simulink model "MultirotorModel_Debugging"  (R2025b)
settings: Solver=ode4  StartTime=0.0  StopTime=350  FixedStep=0.005  RelTol=1e-3  EnableMultiTasking=on
undefined symbols (not defined in the file): angControlTuning, angRateControlTuning, bounds, Controller, decyear, DiscIntNeverNeededParam, DroneMass, dyn_obs, Dz, Gravity, initialConditions, initialGainsMultiplier, Iz, leapyear, max_deviazione_pos, num_rays, Nz, pos_goal, posControlTuning, Pz, startFlightTime, tolleranza_goal, tunePositionController, UAVSampleTime, Vehicle, velControlTuning
libraries: slpidlib x37, slctrl_autotuning x25, sharedutil x4, aerolibconvert2 x3, aerolibatmos2 x2, aerolibgravity2 x2, shared6dof x2, aerolibasang x2, sensorinslib x2, matrix_library x1, uavutilslib x1, uavalgslib x1
(part 6 of 8)

== system MultirotorModel_Debugging/Inner Loop and Plant Model/High-FidelityModel/Control System/Controller/Attitude Controller (autotuning)/Angular Velocity Loop Autotuning ==
  AngVelCtrl_out : Inport
  pitchrollrate_fdbk : Inport  Port=2
  Closed-Loop PID Autotuner : slctrl_autotuning/Closed-Loop PID Autotuner  PIDType=PIDF  PIDForm=Parallel  TimeDomain=discrete-time  DiscreteTs=UAVSampleTime  TuningTs=0.2  UseTuningTs=off  IntegratorFormula=Forward Euler  FilterFormula=Forward Euler  ContinuousTs=0.02  Bandwidth=angRateControlTuning.wc  UseExternalWC=off  TargetPM=angRateControlTuning.pm  UseExternalPM=off  UseExternalAchievedPM=off  ExperimentMode=Superposition  PlantType=Stable  PlantSign=Positive  AmpSine=angRateControlTuning.sineAmp  UseExternalAmpSine=off  UseExternalFRD=off  UseExternalU0=off  UseCompanion=off  NotDeployTuningModule=off  UsePLCCoder=off  OutputMode=perturbation only  BlockDataType=single  UseExperimentGoodPort=off  UseConnectedPID=on  blockpath=[]  tunedP=0  tunedI=0  tunedD=0  tunedN=100  tunedPM=0  EstimationWindowSize=3  UseExternalTuningParams=off  SingleMultiRateVariant=SingleSamplingRate  NumEstimationPeriods=4  NumSettlingPeriods=2  NumOfPRBSPeriod=1  PRBSSignalOrder=12  ExperimentModeVariant=VariantSuperimposed  OutputChoice=VariantDonly  ConvergenceCalcVariant=ConvSuperpositionPRBSVariant
  Closed-Loop PID Autotuner1 : slctrl_autotuning/Closed-Loop PID Autotuner  PIDType=PIDF  PIDForm=Parallel  TimeDomain=discrete-time  DiscreteTs=UAVSampleTime  TuningTs=0.2  UseTuningTs=off  IntegratorFormula=Forward Euler  FilterFormula=Forward Euler  ContinuousTs=0.02  Bandwidth=angRateControlTuning.wc  UseExternalWC=off  TargetPM=angRateControlTuning.pm  UseExternalPM=off  UseExternalAchievedPM=off  ExperimentMode=Superposition  PlantType=Stable  PlantSign=Positive  AmpSine=angRateControlTuning.sineAmp  UseExternalAmpSine=off  UseExternalFRD=off  UseExternalU0=off  UseCompanion=off  NotDeployTuningModule=off  UsePLCCoder=off  OutputMode=perturbation only  BlockDataType=single  UseExperimentGoodPort=off  UseConnectedPID=on  blockpath=[]  tunedP=0  tunedI=0  tunedD=0  tunedN=100  tunedPM=0  EstimationWindowSize=3  UseExternalTuningParams=off  SingleMultiRateVariant=SingleSamplingRate  NumEstimationPeriods=4  NumSettlingPeriods=2  NumOfPRBSPeriod=1  PRBSSignalOrder=12  ExperimentModeVariant=VariantSuperimposed  OutputChoice=VariantDonly  ConvergenceCalcVariant=ConvSuperpositionPRBSVariant
  Display : Display
  Display1 : Display
  Mux : Mux  Inputs=2
  Scope : Scope
      settings: ActiveDisplayYMinimum=99.18257  ActiveDisplayYMaximum=100.62707  DataLoggingVariableName=ScopeData9
  Scope1 : Scope
      settings: DataLoggingVariableName=ScopeData10
  Selector : Selector  InputPortWidth=2  IndexOptions=Index vector (dialog)  Indices=1  OutputSizes=1
  Selector1 : Selector  InputPortWidth=2  IndexOptions=Index vector (dialog)  Indices=1  OutputSizes=1
  Selector2 : Selector  InputPortWidth=2  IndexOptions=Index vector (dialog)  Indices=2  OutputSizes=1
  Selector3 : Selector  InputPortWidth=2  IndexOptions=Index vector (dialog)  Indices=2  OutputSizes=1
  Step : Step  Time=angRateControlTuning.startExpRoll  SampleTime=UAVSampleTime
  Step1 : Step  Time=angRateControlTuning.stopExpRoll  After=-1  SampleTime=UAVSampleTime
  Step2 : Step  Time=angRateControlTuning.startExpPitch  SampleTime=UAVSampleTime
  Step3 : Step  Time=angRateControlTuning.stopExpPitch  After=-1  SampleTime=UAVSampleTime
  Sum : Sum  Inputs=|++
  Sum1 : Sum  Inputs=|++
  Update PID Gains : Subsystem
  pitchrollrate_perturb : Outport
  wires:
  Closed-Loop PID Autotuner1/1 -> Mux/2
  Closed-Loop PID Autotuner1/2 -> Scope1/1
  Sum1/1 -> Update PID Gains/3(start/stop rollrate), Closed-Loop PID Autotuner1/3
  Step/1 -> Sum1/1
  Step1/1 -> Sum1/2
  Selector3/1 -> Closed-Loop PID Autotuner1/2
  Selector2/1 -> Closed-Loop PID Autotuner1/1
  Closed-Loop PID Autotuner/1 -> Mux/1
  Mux/1 -> pitchrollrate_perturb/1
  Closed-Loop PID Autotuner/2 -> Scope/1
  Step3/1 -> Sum/2
  Step2/1 -> Sum/1
  Sum/1 -> Update PID Gains/2(start/stop pitchrate), Closed-Loop PID Autotuner/3
  Selector1/1 -> Closed-Loop PID Autotuner/2
  Selector/1 -> Closed-Loop PID Autotuner/1
  pitchrollrate_fdbk/1 -> Selector1/1, Selector3/1
  AngVelCtrl_out/1 -> Selector/1, Selector2/1
  Closed-Loop PID Autotuner/3 -> Update PID Gains/1(PID Gains pitchrate), Display/1
  Closed-Loop PID Autotuner1/3 -> Update PID Gains/4(PID Gains rollrate), Display1/1

== system MultirotorModel_Debugging/Inner Loop and Plant Model/High-FidelityModel/Control System/Controller/Position Controller (autotuning)/Position Loop Autotuning ==
  PosCtrl_out : Inport
  xy_fdbk : Inport  Port=2
  Closed-Loop PID Autotuner : slctrl_autotuning/Closed-Loop PID Autotuner  PIDType=P  PIDForm=Parallel  TimeDomain=discrete-time  DiscreteTs=UAVSampleTime  TuningTs=0.2  UseTuningTs=off  IntegratorFormula=Forward Euler  FilterFormula=Forward Euler  ContinuousTs=0.02  Bandwidth=posControlTuning.wc  UseExternalWC=off  TargetPM=posControlTuning.pm  UseExternalPM=off  UseExternalAchievedPM=off  ExperimentMode=Superposition  PlantType=Stable  PlantSign=Positive  AmpSine=posControlTuning.sineAmp  UseExternalAmpSine=off  UseExternalFRD=off  UseExternalU0=off  UseCompanion=off  NotDeployTuningModule=off  UsePLCCoder=off  OutputMode=perturbation only  BlockDataType=single  UseExperimentGoodPort=off  UseConnectedPID=on  blockpath=[]  tunedP=0  tunedI=0  tunedD=0  tunedN=100  tunedPM=0  EstimationWindowSize=3  UseExternalTuningParams=off  SingleMultiRateVariant=SingleSamplingRate  NumEstimationPeriods=4  NumSettlingPeriods=2  NumOfPRBSPeriod=1  PRBSSignalOrder=12  ExperimentModeVariant=VariantSuperimposed  OutputChoice=VariantDonly  ConvergenceCalcVariant=ConvSuperpositionPRBSVariant
  Closed-Loop PID Autotuner1 : slctrl_autotuning/Closed-Loop PID Autotuner  PIDType=P  PIDForm=Parallel  TimeDomain=discrete-time  DiscreteTs=UAVSampleTime  TuningTs=0.2  UseTuningTs=off  IntegratorFormula=Forward Euler  FilterFormula=Forward Euler  ContinuousTs=0.02  Bandwidth=posControlTuning.wc  UseExternalWC=off  TargetPM=posControlTuning.pm  UseExternalPM=off  UseExternalAchievedPM=off  ExperimentMode=Superposition  PlantType=Stable  PlantSign=Positive  AmpSine=posControlTuning.sineAmp  UseExternalAmpSine=off  UseExternalFRD=off  UseExternalU0=off  UseCompanion=off  NotDeployTuningModule=off  UsePLCCoder=off  OutputMode=perturbation only  BlockDataType=single  UseExperimentGoodPort=off  UseConnectedPID=on  blockpath=[]  tunedP=0  tunedI=0  tunedD=0  tunedN=100  tunedPM=0  EstimationWindowSize=3  UseExternalTuningParams=off  SingleMultiRateVariant=SingleSamplingRate  NumEstimationPeriods=4  NumSettlingPeriods=2  NumOfPRBSPeriod=1  PRBSSignalOrder=12  ExperimentModeVariant=VariantSuperimposed  OutputChoice=VariantDonly  ConvergenceCalcVariant=ConvSuperpositionPRBSVariant
  Display : Display
  Display1 : Display
  Gain1 : Gain  Gain=tunePositionController
  Gain2 : Gain  Gain=tunePositionController
  Mux : Mux  Inputs=2
  Selector : Selector  InputPortWidth=2  IndexOptions=Index vector (dialog)  Indices=1  OutputSizes=1
  Selector1 : Selector  InputPortWidth=2  IndexOptions=Index vector (dialog)  Indices=1  OutputSizes=1
  Selector2 : Selector  InputPortWidth=2  IndexOptions=Index vector (dialog)  Indices=2  OutputSizes=1
  Selector3 : Selector  InputPortWidth=2  IndexOptions=Index vector (dialog)  Indices=2  OutputSizes=1
  Step : Step  Time=posControlTuning.startExpX  SampleTime=UAVSampleTime
  Step1 : Step  Time=posControlTuning.stopExpX  After=-1  SampleTime=UAVSampleTime
  Step2 : Step  Time=posControlTuning.startExpY  SampleTime=UAVSampleTime
  Step3 : Step  Time=posControlTuning.stopExpY  After=-1  SampleTime=UAVSampleTime
  Sum : Sum  Inputs=|++
  Sum1 : Sum  Inputs=|++
  Terminator : Terminator
  Terminator1 : Terminator
  Update PID Gains : Subsystem
  xy_perturb : Outport
  wires:
  PosCtrl_out/1 -> Selector2/1, Selector/1
  xy_fdbk/1 -> Selector3/1, Selector1/1
  Selector/1 -> Closed-Loop PID Autotuner/1
  Selector1/1 -> Closed-Loop PID Autotuner/2
  Sum/1 -> Gain1/1
  Step/1 -> Sum/1
  Step1/1 -> Sum/2
  Closed-Loop PID Autotuner/2 -> Terminator/1
  Mux/1 -> xy_perturb/1
  Closed-Loop PID Autotuner/1 -> Mux/1
  Selector2/1 -> Closed-Loop PID Autotuner1/1
  Selector3/1 -> Closed-Loop PID Autotuner1/2
  Step3/1 -> Sum1/2
  Step2/1 -> Sum1/1
  Sum1/1 -> Gain2/1
  Closed-Loop PID Autotuner1/2 -> Terminator1/1
  Closed-Loop PID Autotuner1/1 -> Mux/2
  Closed-Loop PID Autotuner/3 -> Update PID Gains/1(PID Gains X), Display/1
  Closed-Loop PID Autotuner1/3 -> Update PID Gains/4(PID Gains Y), Display1/1
  Gain1/1 -> Update PID Gains/2(start/stop X), Closed-Loop PID Autotuner/3
  Gain2/1 -> Update PID Gains/3(start/stop Y), Closed-Loop PID Autotuner1/3

== system MultirotorModel_Debugging/Inner Loop and Plant Model/High-FidelityModel/Control System/Controller/Position Controller (autotuning)/Velocity Loop Autotuning ==
  VelCtrl_out : Inport
  xxyy_fdbk : Inport  Port=2
  Closed-Loop PID Autotuner : slctrl_autotuning/Closed-Loop PID Autotuner  PIDType=PI  PIDForm=Parallel  TimeDomain=discrete-time  DiscreteTs=UAVSampleTime  TuningTs=0.2  UseTuningTs=off  IntegratorFormula=Forward Euler  FilterFormula=Forward Euler  ContinuousTs=0.02  Bandwidth=velControlTuning.wc  UseExternalWC=off  TargetPM=velControlTuning.pm  UseExternalPM=off  UseExternalAchievedPM=off  ExperimentMode=Superposition  PlantType=Stable  PlantSign=Positive  AmpSine=velControlTuning.sineAmp  UseExternalAmpSine=off  UseExternalFRD=off  UseExternalU0=off  UseCompanion=off  NotDeployTuningModule=off  UsePLCCoder=off  OutputMode=perturbation only  BlockDataType=single  UseExperimentGoodPort=off  UseConnectedPID=on  blockpath=[]  tunedP=0  tunedI=0  tunedD=0  tunedN=100  tunedPM=0  EstimationWindowSize=3  UseExternalTuningParams=off  SingleMultiRateVariant=SingleSamplingRate  NumEstimationPeriods=4  NumSettlingPeriods=2  NumOfPRBSPeriod=1  PRBSSignalOrder=12  ExperimentModeVariant=VariantSuperimposed  OutputChoice=VariantDonly  ConvergenceCalcVariant=ConvSuperpositionPRBSVariant
  Closed-Loop PID Autotuner1 : slctrl_autotuning/Closed-Loop PID Autotuner  PIDType=PI  PIDForm=Parallel  TimeDomain=discrete-time  DiscreteTs=UAVSampleTime  TuningTs=0.2  UseTuningTs=off  IntegratorFormula=Forward Euler  FilterFormula=Forward Euler  ContinuousTs=0.02  Bandwidth=velControlTuning.wc  UseExternalWC=off  TargetPM=velControlTuning.pm  UseExternalPM=off  UseExternalAchievedPM=off  ExperimentMode=Superposition  PlantType=Stable  PlantSign=Positive  AmpSine=velControlTuning.sineAmp  UseExternalAmpSine=off  UseExternalFRD=off  UseExternalU0=off  UseCompanion=off  NotDeployTuningModule=off  UsePLCCoder=off  OutputMode=perturbation only  BlockDataType=single  UseExperimentGoodPort=off  UseConnectedPID=on  blockpath=[]  tunedP=0  tunedI=0  tunedD=0  tunedN=100  tunedPM=0  EstimationWindowSize=3  UseExternalTuningParams=off  SingleMultiRateVariant=SingleSamplingRate  NumEstimationPeriods=4  NumSettlingPeriods=2  NumOfPRBSPeriod=1  PRBSSignalOrder=12  ExperimentModeVariant=VariantSuperimposed  OutputChoice=VariantDonly  ConvergenceCalcVariant=ConvSuperpositionPRBSVariant
  Display : Display
  Display1 : Display
  Gain : Gain  Gain=tunePositionController
  Gain1 : Gain  Gain=tunePositionController
  Mux : Mux  Inputs=2
  Scope : Scope
      settings: ActiveDisplayYMinimum=99.18257  ActiveDisplayYMaximum=100.62707  DataLoggingVariableName=ScopeData9
  Scope1 : Scope
      settings: DataLoggingVariableName=ScopeData10
  Selector : Selector  InputPortWidth=2  IndexOptions=Index vector (dialog)  Indices=1  OutputSizes=1
  Selector1 : Selector  InputPortWidth=2  IndexOptions=Index vector (dialog)  Indices=1  OutputSizes=1
  Selector2 : Selector  InputPortWidth=2  IndexOptions=Index vector (dialog)  Indices=2  OutputSizes=1
  Selector3 : Selector  InputPortWidth=2  IndexOptions=Index vector (dialog)  Indices=2  OutputSizes=1
  Step : Step  Time=velControlTuning.startExpX  SampleTime=UAVSampleTime
  Step1 : Step  Time=velControlTuning.stopExpX  After=-1  SampleTime=UAVSampleTime
  Step2 : Step  Time=velControlTuning.startExpY  SampleTime=UAVSampleTime
  Step3 : Step  Time=velControlTuning.stopExpY  After=-1  SampleTime=UAVSampleTime
  Sum : Sum  Inputs=|++
  Sum1 : Sum  Inputs=|++
  Update PID Gains : Subsystem
  xxyy_perturb : Outport
  wires:
  Closed-Loop PID Autotuner1/1 -> Mux/2
  Closed-Loop PID Autotuner1/2 -> Scope1/1
  Sum1/1 -> Gain1/1
  Step2/1 -> Sum1/1
  Step3/1 -> Sum1/2
  Selector3/1 -> Closed-Loop PID Autotuner1/2
  Selector2/1 -> Closed-Loop PID Autotuner1/1
  Closed-Loop PID Autotuner/1 -> Mux/1
  Mux/1 -> xxyy_perturb/1
  Closed-Loop PID Autotuner/2 -> Scope/1
  Step1/1 -> Sum/2
  Step/1 -> Sum/1
  Sum/1 -> Gain/1
  Selector1/1 -> Closed-Loop PID Autotuner/2
  Selector/1 -> Closed-Loop PID Autotuner/1
  xxyy_fdbk/1 -> Selector1/1, Selector3/1
  VelCtrl_out/1 -> Selector/1, Selector2/1
  Closed-Loop PID Autotuner/3 -> Update PID Gains/1(PID Gains XX), Display/1
  Closed-Loop PID Autotuner1/3 -> Update PID Gains/4(PID Gains YY), Display1/1
  Gain/1 -> Update PID Gains/2(start/stop XX), Closed-Loop PID Autotuner/3
  Gain1/1 -> Update PID Gains/3(start/stop YY), Closed-Loop PID Autotuner1/3

== system MultirotorModel_Debugging/Inner Loop and Plant Model/High-FidelityModel/Control System/Controller/Position Controller (autotuning, solo vel)/Position Loop Autotuning ==
  PosCtrl_out : Inport
  xy_fdbk : Inport  Port=2
  Closed-Loop PID Autotuner : slctrl_autotuning/Closed-Loop PID Autotuner  PIDType=P  PIDForm=Parallel  TimeDomain=discrete-time  DiscreteTs=UAVSampleTime  TuningTs=0.2  UseTuningTs=off  IntegratorFormula=Forward Euler  FilterFormula=Forward Euler  ContinuousTs=0.02  Bandwidth=posControlTuning.wc  UseExternalWC=off  TargetPM=posControlTuning.pm  UseExternalPM=off  UseExternalAchievedPM=off  ExperimentMode=Superposition  PlantType=Stable  PlantSign=Positive  AmpSine=posControlTuning.sineAmp  UseExternalAmpSine=off  UseExternalFRD=off  UseExternalU0=off  UseCompanion=off  NotDeployTuningModule=off  UsePLCCoder=off  OutputMode=perturbation only  BlockDataType=single  UseExperimentGoodPort=off  UseConnectedPID=on  blockpath=[]  tunedP=0  tunedI=0  tunedD=0  tunedN=100  tunedPM=0  EstimationWindowSize=3  UseExternalTuningParams=off  SingleMultiRateVariant=SingleSamplingRate  NumEstimationPeriods=4  NumSettlingPeriods=2  NumOfPRBSPeriod=1  PRBSSignalOrder=12  ExperimentModeVariant=VariantSuperimposed  OutputChoice=VariantDonly  ConvergenceCalcVariant=ConvSuperpositionPRBSVariant
  Closed-Loop PID Autotuner1 : slctrl_autotuning/Closed-Loop PID Autotuner  PIDType=P  PIDForm=Parallel  TimeDomain=discrete-time  DiscreteTs=UAVSampleTime  TuningTs=0.2  UseTuningTs=off  IntegratorFormula=Forward Euler  FilterFormula=Forward Euler  ContinuousTs=0.02  Bandwidth=posControlTuning.wc  UseExternalWC=off  TargetPM=posControlTuning.pm  UseExternalPM=off  UseExternalAchievedPM=off  ExperimentMode=Superposition  PlantType=Stable  PlantSign=Positive  AmpSine=posControlTuning.sineAmp  UseExternalAmpSine=off  UseExternalFRD=off  UseExternalU0=off  UseCompanion=off  NotDeployTuningModule=off  UsePLCCoder=off  OutputMode=perturbation only  BlockDataType=single  UseExperimentGoodPort=off  UseConnectedPID=on  blockpath=[]  tunedP=0  tunedI=0  tunedD=0  tunedN=100  tunedPM=0  EstimationWindowSize=3  UseExternalTuningParams=off  SingleMultiRateVariant=SingleSamplingRate  NumEstimationPeriods=4  NumSettlingPeriods=2  NumOfPRBSPeriod=1  PRBSSignalOrder=12  ExperimentModeVariant=VariantSuperimposed  OutputChoice=VariantDonly  ConvergenceCalcVariant=ConvSuperpositionPRBSVariant
  Display : Display
  Display1 : Display
  Gain1 : Gain  Gain=tunePositionController
  Gain2 : Gain  Gain=tunePositionController
  Mux : Mux  Inputs=2
  Selector : Selector  InputPortWidth=2  IndexOptions=Index vector (dialog)  Indices=1  OutputSizes=1
  Selector1 : Selector  InputPortWidth=2  IndexOptions=Index vector (dialog)  Indices=1  OutputSizes=1
  Selector2 : Selector  InputPortWidth=2  IndexOptions=Index vector (dialog)  Indices=2  OutputSizes=1
  Selector3 : Selector  InputPortWidth=2  IndexOptions=Index vector (dialog)  Indices=2  OutputSizes=1
  Step : Step  Time=posControlTuning.startExpX  SampleTime=UAVSampleTime
  Step1 : Step  Time=posControlTuning.stopExpX  After=-1  SampleTime=UAVSampleTime
  Step2 : Step  Time=posControlTuning.startExpY  SampleTime=UAVSampleTime
  Step3 : Step  Time=posControlTuning.stopExpY  After=-1  SampleTime=UAVSampleTime
  Sum : Sum  Inputs=|++
  Sum1 : Sum  Inputs=|++
  Terminator : Terminator
  Terminator1 : Terminator
  Update PID Gains : Subsystem
  xy_perturb : Outport
  wires:
  PosCtrl_out/1 -> Selector2/1, Selector/1
  xy_fdbk/1 -> Selector3/1, Selector1/1
  Selector/1 -> Closed-Loop PID Autotuner/1
  Selector1/1 -> Closed-Loop PID Autotuner/2
  Sum/1 -> Gain1/1
  Step/1 -> Sum/1
  Step1/1 -> Sum/2
  Closed-Loop PID Autotuner/2 -> Terminator/1
  Mux/1 -> xy_perturb/1
  Closed-Loop PID Autotuner/1 -> Mux/1
  Selector2/1 -> Closed-Loop PID Autotuner1/1
  Selector3/1 -> Closed-Loop PID Autotuner1/2
  Step3/1 -> Sum1/2
  Step2/1 -> Sum1/1
  Sum1/1 -> Gain2/1
  Closed-Loop PID Autotuner1/2 -> Terminator1/1
  Closed-Loop PID Autotuner1/1 -> Mux/2
  Closed-Loop PID Autotuner/3 -> Update PID Gains/1(PID Gains X), Display/1
  Closed-Loop PID Autotuner1/3 -> Update PID Gains/4(PID Gains Y), Display1/1
  Gain1/1 -> Update PID Gains/2(start/stop X), Closed-Loop PID Autotuner/3
  Gain2/1 -> Update PID Gains/3(start/stop Y), Closed-Loop PID Autotuner1/3

== system MultirotorModel_Debugging/Inner Loop and Plant Model/High-FidelityModel/Control System/Controller/Position Controller (autotuning, solo vel)/Velocity Loop Autotuning ==
  VelCtrl_out : Inport
  xxyy_fdbk : Inport  Port=2
  Closed-Loop PID Autotuner : slctrl_autotuning/Closed-Loop PID Autotuner  PIDType=PI  PIDForm=Parallel  TimeDomain=discrete-time  DiscreteTs=UAVSampleTime  TuningTs=0.2  UseTuningTs=off  IntegratorFormula=Forward Euler  FilterFormula=Forward Euler  ContinuousTs=0.02  Bandwidth=velControlTuning.wc  UseExternalWC=off  TargetPM=velControlTuning.pm  UseExternalPM=off  UseExternalAchievedPM=off  ExperimentMode=Superposition  PlantType=Stable  PlantSign=Positive  AmpSine=velControlTuning.sineAmp  UseExternalAmpSine=off  UseExternalFRD=off  UseExternalU0=off  UseCompanion=off  NotDeployTuningModule=off  UsePLCCoder=off  OutputMode=perturbation only  BlockDataType=single  UseExperimentGoodPort=off  UseConnectedPID=on  blockpath=[]  tunedP=0  tunedI=0  tunedD=0  tunedN=100  tunedPM=0  EstimationWindowSize=3  UseExternalTuningParams=off  SingleMultiRateVariant=SingleSamplingRate  NumEstimationPeriods=4  NumSettlingPeriods=2  NumOfPRBSPeriod=1  PRBSSignalOrder=12  ExperimentModeVariant=VariantSuperimposed  OutputChoice=VariantDonly  ConvergenceCalcVariant=ConvSuperpositionPRBSVariant
  Closed-Loop PID Autotuner1 : slctrl_autotuning/Closed-Loop PID Autotuner  PIDType=PI  PIDForm=Parallel  TimeDomain=discrete-time  DiscreteTs=UAVSampleTime  TuningTs=0.2  UseTuningTs=off  IntegratorFormula=Forward Euler  FilterFormula=Forward Euler  ContinuousTs=0.02  Bandwidth=velControlTuning.wc  UseExternalWC=off  TargetPM=velControlTuning.pm  UseExternalPM=off  UseExternalAchievedPM=off  ExperimentMode=Superposition  PlantType=Stable  PlantSign=Positive  AmpSine=velControlTuning.sineAmp  UseExternalAmpSine=off  UseExternalFRD=off  UseExternalU0=off  UseCompanion=off  NotDeployTuningModule=off  UsePLCCoder=off  OutputMode=perturbation only  BlockDataType=single  UseExperimentGoodPort=off  UseConnectedPID=on  blockpath=[]  tunedP=0  tunedI=0  tunedD=0  tunedN=100  tunedPM=0  EstimationWindowSize=3  UseExternalTuningParams=off  SingleMultiRateVariant=SingleSamplingRate  NumEstimationPeriods=4  NumSettlingPeriods=2  NumOfPRBSPeriod=1  PRBSSignalOrder=12  ExperimentModeVariant=VariantSuperimposed  OutputChoice=VariantDonly  ConvergenceCalcVariant=ConvSuperpositionPRBSVariant
  Display : Display
  Display1 : Display
  Gain : Gain  Gain=tunePositionController
  Gain1 : Gain  Gain=tunePositionController
  Mux : Mux  Inputs=2
  Scope : Scope
      settings: ActiveDisplayYMinimum=99.18257  ActiveDisplayYMaximum=100.62707  DataLoggingVariableName=ScopeData9
  Scope1 : Scope
      settings: DataLoggingVariableName=ScopeData10
  Selector : Selector  InputPortWidth=2  IndexOptions=Index vector (dialog)  Indices=1  OutputSizes=1
  Selector1 : Selector  InputPortWidth=2  IndexOptions=Index vector (dialog)  Indices=1  OutputSizes=1
  Selector2 : Selector  InputPortWidth=2  IndexOptions=Index vector (dialog)  Indices=2  OutputSizes=1
  Selector3 : Selector  InputPortWidth=2  IndexOptions=Index vector (dialog)  Indices=2  OutputSizes=1
  Step : Step  Time=velControlTuning.startExpX  SampleTime=UAVSampleTime
  Step1 : Step  Time=velControlTuning.stopExpX  After=-1  SampleTime=UAVSampleTime
  Step2 : Step  Time=velControlTuning.startExpY  SampleTime=UAVSampleTime
  Step3 : Step  Time=velControlTuning.stopExpY  After=-1  SampleTime=UAVSampleTime
  Sum : Sum  Inputs=|++
  Sum1 : Sum  Inputs=|++
  Update PID Gains : Subsystem
  xxyy_perturb : Outport
  wires:
  Closed-Loop PID Autotuner1/1 -> Mux/2
  Closed-Loop PID Autotuner1/2 -> Scope1/1
  Sum1/1 -> Gain1/1
  Step2/1 -> Sum1/1
  Step3/1 -> Sum1/2
  Selector3/1 -> Closed-Loop PID Autotuner1/2
  Selector2/1 -> Closed-Loop PID Autotuner1/1
  Closed-Loop PID Autotuner/1 -> Mux/1
  Mux/1 -> xxyy_perturb/1
  Closed-Loop PID Autotuner/2 -> Scope/1
  Step1/1 -> Sum/2
  Step/1 -> Sum/1
  Sum/1 -> Gain/1
  Selector1/1 -> Closed-Loop PID Autotuner/2
  Selector/1 -> Closed-Loop PID Autotuner/1
  xxyy_fdbk/1 -> Selector1/1, Selector3/1
  VelCtrl_out/1 -> Selector/1, Selector2/1
  Closed-Loop PID Autotuner/3 -> Update PID Gains/1(PID Gains XX), Display/1
  Closed-Loop PID Autotuner1/3 -> Update PID Gains/4(PID Gains YY), Display1/1
  Gain/1 -> Update PID Gains/2(start/stop XX), Closed-Loop PID Autotuner/3
  Gain1/1 -> Update PID Gains/3(start/stop YY), Closed-Loop PID Autotuner1/3

== system MultirotorModel_Debugging/Inner Loop and Plant Model/High-FidelityModel/Control System/Controller/Position Controller 3 (autotuning, vel + pos)/Position Loop Autotuning ==
  PosCtrl_out : Inport
  xy_fdbk : Inport  Port=2
  Closed-Loop PID Autotuner : slctrl_autotuning/Closed-Loop PID Autotuner  PIDType=P  PIDForm=Parallel  TimeDomain=discrete-time  DiscreteTs=UAVSampleTime  TuningTs=0.2  UseTuningTs=off  IntegratorFormula=Forward Euler  FilterFormula=Forward Euler  ContinuousTs=0.02  Bandwidth=posControlTuning.wc  UseExternalWC=off  TargetPM=posControlTuning.pm  UseExternalPM=off  UseExternalAchievedPM=off  ExperimentMode=Superposition  PlantType=Stable  PlantSign=Positive  AmpSine=posControlTuning.sineAmp  UseExternalAmpSine=off  UseExternalFRD=off  UseExternalU0=off  UseCompanion=off  NotDeployTuningModule=off  UsePLCCoder=off  OutputMode=perturbation only  BlockDataType=single  UseExperimentGoodPort=off  UseConnectedPID=on  blockpath=[]  tunedP=0  tunedI=0  tunedD=0  tunedN=100  tunedPM=0  EstimationWindowSize=3  UseExternalTuningParams=off  SingleMultiRateVariant=SingleSamplingRate  NumEstimationPeriods=4  NumSettlingPeriods=2  NumOfPRBSPeriod=1  PRBSSignalOrder=12  ExperimentModeVariant=VariantSuperimposed  OutputChoice=VariantDonly  ConvergenceCalcVariant=ConvSuperpositionPRBSVariant
  Closed-Loop PID Autotuner1 : slctrl_autotuning/Closed-Loop PID Autotuner  PIDType=P  PIDForm=Parallel  TimeDomain=discrete-time  DiscreteTs=UAVSampleTime  TuningTs=0.2  UseTuningTs=off  IntegratorFormula=Forward Euler  FilterFormula=Forward Euler  ContinuousTs=0.02  Bandwidth=posControlTuning.wc  UseExternalWC=off  TargetPM=posControlTuning.pm  UseExternalPM=off  UseExternalAchievedPM=off  ExperimentMode=Superposition  PlantType=Stable  PlantSign=Positive  AmpSine=posControlTuning.sineAmp  UseExternalAmpSine=off  UseExternalFRD=off  UseExternalU0=off  UseCompanion=off  NotDeployTuningModule=off  UsePLCCoder=off  OutputMode=perturbation only  BlockDataType=single  UseExperimentGoodPort=off  UseConnectedPID=on  blockpath=[]  tunedP=0  tunedI=0  tunedD=0  tunedN=100  tunedPM=0  EstimationWindowSize=3  UseExternalTuningParams=off  SingleMultiRateVariant=SingleSamplingRate  NumEstimationPeriods=4  NumSettlingPeriods=2  NumOfPRBSPeriod=1  PRBSSignalOrder=12  ExperimentModeVariant=VariantSuperimposed  OutputChoice=VariantDonly  ConvergenceCalcVariant=ConvSuperpositionPRBSVariant
  Display : Display
  Display1 : Display
  Gain1 : Gain  Gain=tunePositionController
  Gain2 : Gain  Gain=tunePositionController
  Mux : Mux  Inputs=2
  Selector : Selector  InputPortWidth=2  IndexOptions=Index vector (dialog)  Indices=1  OutputSizes=1
  Selector1 : Selector  InputPortWidth=2  IndexOptions=Index vector (dialog)  Indices=1  OutputSizes=1
  Selector2 : Selector  InputPortWidth=2  IndexOptions=Index vector (dialog)  Indices=2  OutputSizes=1
  Selector3 : Selector  InputPortWidth=2  IndexOptions=Index vector (dialog)  Indices=2  OutputSizes=1
  Step : Step  Time=posControlTuning.startExpX  SampleTime=UAVSampleTime
  Step1 : Step  Time=posControlTuning.stopExpX  After=-1  SampleTime=UAVSampleTime
  Step2 : Step  Time=posControlTuning.startExpY  SampleTime=UAVSampleTime
  Step3 : Step  Time=posControlTuning.stopExpY  After=-1  SampleTime=UAVSampleTime
  Sum : Sum  Inputs=|++
  Sum1 : Sum  Inputs=|++
  Terminator : Terminator
  Terminator1 : Terminator
  Update PID Gains : Subsystem
  xy_perturb : Outport
  wires:
  PosCtrl_out/1 -> Selector2/1, Selector/1
  xy_fdbk/1 -> Selector3/1, Selector1/1
  Selector/1 -> Closed-Loop PID Autotuner/1
  Selector1/1 -> Closed-Loop PID Autotuner/2
  Sum/1 -> Gain1/1
  Step/1 -> Sum/1
  Step1/1 -> Sum/2
  Closed-Loop PID Autotuner/2 -> Terminator/1
  Mux/1 -> xy_perturb/1
  Closed-Loop PID Autotuner/1 -> Mux/1
  Selector2/1 -> Closed-Loop PID Autotuner1/1
  Selector3/1 -> Closed-Loop PID Autotuner1/2
  Step3/1 -> Sum1/2
  Step2/1 -> Sum1/1
  Sum1/1 -> Gain2/1
  Closed-Loop PID Autotuner1/2 -> Terminator1/1
  Closed-Loop PID Autotuner1/1 -> Mux/2
  Closed-Loop PID Autotuner/3 -> Update PID Gains/1(PID Gains X), Display/1
  Closed-Loop PID Autotuner1/3 -> Update PID Gains/4(PID Gains Y), Display1/1
  Gain1/1 -> Update PID Gains/2(start/stop X), Closed-Loop PID Autotuner/3
  Gain2/1 -> Update PID Gains/3(start/stop Y), Closed-Loop PID Autotuner1/3

== system MultirotorModel_Debugging/Inner Loop and Plant Model/High-FidelityModel/Control System/Controller/Position Controller 3 (autotuning, vel + pos)/Velocity Loop Autotuning ==
  VelCtrl_out : Inport
  xxyy_fdbk : Inport  Port=2
  Closed-Loop PID Autotuner : slctrl_autotuning/Closed-Loop PID Autotuner  PIDType=PI  PIDForm=Parallel  TimeDomain=discrete-time  DiscreteTs=UAVSampleTime  TuningTs=0.2  UseTuningTs=off  IntegratorFormula=Forward Euler  FilterFormula=Forward Euler  ContinuousTs=0.02  Bandwidth=velControlTuning.wc  UseExternalWC=off  TargetPM=velControlTuning.pm  UseExternalPM=off  UseExternalAchievedPM=off  ExperimentMode=Superposition  PlantType=Stable  PlantSign=Positive  AmpSine=velControlTuning.sineAmp  UseExternalAmpSine=off  UseExternalFRD=off  UseExternalU0=off  UseCompanion=off  NotDeployTuningModule=off  UsePLCCoder=off  OutputMode=perturbation only  BlockDataType=single  UseExperimentGoodPort=off  UseConnectedPID=on  blockpath=[]  tunedP=0  tunedI=0  tunedD=0  tunedN=100  tunedPM=0  EstimationWindowSize=3  UseExternalTuningParams=off  SingleMultiRateVariant=SingleSamplingRate  NumEstimationPeriods=4  NumSettlingPeriods=2  NumOfPRBSPeriod=1  PRBSSignalOrder=12  ExperimentModeVariant=VariantSuperimposed  OutputChoice=VariantDonly  ConvergenceCalcVariant=ConvSuperpositionPRBSVariant
  Closed-Loop PID Autotuner1 : slctrl_autotuning/Closed-Loop PID Autotuner  PIDType=PI  PIDForm=Parallel  TimeDomain=discrete-time  DiscreteTs=UAVSampleTime  TuningTs=0.2  UseTuningTs=off  IntegratorFormula=Forward Euler  FilterFormula=Forward Euler  ContinuousTs=0.02  Bandwidth=velControlTuning.wc  UseExternalWC=off  TargetPM=velControlTuning.pm  UseExternalPM=off  UseExternalAchievedPM=off  ExperimentMode=Superposition  PlantType=Stable  PlantSign=Positive  AmpSine=velControlTuning.sineAmp  UseExternalAmpSine=off  UseExternalFRD=off  UseExternalU0=off  UseCompanion=off  NotDeployTuningModule=off  UsePLCCoder=off  OutputMode=perturbation only  BlockDataType=single  UseExperimentGoodPort=off  UseConnectedPID=on  blockpath=[]  tunedP=0  tunedI=0  tunedD=0  tunedN=100  tunedPM=0  EstimationWindowSize=3  UseExternalTuningParams=off  SingleMultiRateVariant=SingleSamplingRate  NumEstimationPeriods=4  NumSettlingPeriods=2  NumOfPRBSPeriod=1  PRBSSignalOrder=12  ExperimentModeVariant=VariantSuperimposed  OutputChoice=VariantDonly  ConvergenceCalcVariant=ConvSuperpositionPRBSVariant
  Display : Display
  Display1 : Display
  Gain : Gain  Gain=tunePositionController
  Gain1 : Gain  Gain=tunePositionController
  Mux : Mux  Inputs=2
  Scope : Scope
      settings: ActiveDisplayYMinimum=99.18257  ActiveDisplayYMaximum=100.62707  DataLoggingVariableName=ScopeData9
  Scope1 : Scope
      settings: DataLoggingVariableName=ScopeData10
  Selector : Selector  InputPortWidth=2  IndexOptions=Index vector (dialog)  Indices=1  OutputSizes=1
  Selector1 : Selector  InputPortWidth=2  IndexOptions=Index vector (dialog)  Indices=1  OutputSizes=1
  Selector2 : Selector  InputPortWidth=2  IndexOptions=Index vector (dialog)  Indices=2  OutputSizes=1
  Selector3 : Selector  InputPortWidth=2  IndexOptions=Index vector (dialog)  Indices=2  OutputSizes=1
  Step : Step  Time=velControlTuning.startExpX  SampleTime=UAVSampleTime
  Step1 : Step  Time=velControlTuning.stopExpX  After=-1  SampleTime=UAVSampleTime
  Step2 : Step  Time=velControlTuning.startExpY  SampleTime=UAVSampleTime
  Step3 : Step  Time=velControlTuning.stopExpY  After=-1  SampleTime=UAVSampleTime
  Sum : Sum  Inputs=|++
  Sum1 : Sum  Inputs=|++
  Update PID Gains : Subsystem
  xxyy_perturb : Outport
  wires:
  Closed-Loop PID Autotuner1/1 -> Mux/2
  Closed-Loop PID Autotuner1/2 -> Scope1/1
  Sum1/1 -> Gain1/1
  Step2/1 -> Sum1/1
  Step3/1 -> Sum1/2
  Selector3/1 -> Closed-Loop PID Autotuner1/2
  Selector2/1 -> Closed-Loop PID Autotuner1/1
  Closed-Loop PID Autotuner/1 -> Mux/1
  Mux/1 -> xxyy_perturb/1
  Closed-Loop PID Autotuner/2 -> Scope/1
  Step1/1 -> Sum/2
  Step/1 -> Sum/1
  Sum/1 -> Gain/1
  Selector1/1 -> Closed-Loop PID Autotuner/2
  Selector/1 -> Closed-Loop PID Autotuner/1
  xxyy_fdbk/1 -> Selector1/1, Selector3/1
  VelCtrl_out/1 -> Selector/1, Selector2/1
  Closed-Loop PID Autotuner/3 -> Update PID Gains/1(PID Gains XX), Display/1
  Closed-Loop PID Autotuner1/3 -> Update PID Gains/4(PID Gains YY), Display1/1
  Gain/1 -> Update PID Gains/2(start/stop XX), Closed-Loop PID Autotuner/3
  Gain1/1 -> Update PID Gains/3(start/stop YY), Closed-Loop PID Autotuner1/3

== system MultirotorModel_Debugging/Inner Loop and Plant Model/High-FidelityModel/Control System/Controller/gravity feedforward//equilibrium thrust (autotuning)/Angular Velocity Loop Autotuning ==
  Altitude_out : Inport
  z_fdbk : Inport  Port=2
  Closed-Loop PID Autotuner : slctrl_autotuning/Closed-Loop PID Autotuner  PIDType=PIDF  PIDForm=Parallel  TimeDomain=discrete-time  DiscreteTs=UAVSampleTime  TuningTs=0.2  UseTuningTs=off  IntegratorFormula=Forward Euler  FilterFormula=Forward Euler  ContinuousTs=0.02  Bandwidth=angRateControlTuning.wc  UseExternalWC=off  TargetPM=angRateControlTuning.pm  UseExternalPM=off  UseExternalAchievedPM=off  ExperimentMode=Superposition  PlantType=Stable  PlantSign=Positive  AmpSine=angRateControlTuning.sineAmp  UseExternalAmpSine=off  UseExternalFRD=off  UseExternalU0=off  UseCompanion=off  NotDeployTuningModule=off  UsePLCCoder=off  OutputMode=perturbation only  BlockDataType=single  UseExperimentGoodPort=off  UseConnectedPID=on  blockpath=[]  tunedP=0  tunedI=0  tunedD=0  tunedN=100  tunedPM=0  EstimationWindowSize=3  UseExternalTuningParams=off  SingleMultiRateVariant=SingleSamplingRate  NumEstimationPeriods=4  NumSettlingPeriods=2  NumOfPRBSPeriod=1  PRBSSignalOrder=12  ExperimentModeVariant=VariantSuperimposed  OutputChoice=VariantDonly  ConvergenceCalcVariant=ConvSuperpositionPRBSVariant
  Display : Display
  Gain1 : Gain  Gain=tunePositionController
  Scope : Scope
      settings: ActiveDisplayYMinimum=99.18257  ActiveDisplayYMaximum=100.62707  DataLoggingVariableName=ScopeData9
  Step : Step  Time=posControlTuning.startExpX  SampleTime=UAVSampleTime
  Step1 : Step  Time=posControlTuning.stopExpX  After=-1  SampleTime=UAVSampleTime
  Sum : Sum  Inputs=|++
  Unit Delay2 : UnitDelay  SampleTime=UAVSampleTime  HasFrameUpgradeWarning=on
  Update PID Gains Z : Subsystem
  z_perturb : Outport
  wires:
  Closed-Loop PID Autotuner/1 -> z_perturb/1
  Closed-Loop PID Autotuner/2 -> Scope/1
  z_fdbk/1 -> Closed-Loop PID Autotuner/2
  Altitude_out/1 -> Closed-Loop PID Autotuner/1
  Unit Delay2/1 -> Update PID Gains Z/Trigger
  Gain1/1 -> Unit Delay2/1, Closed-Loop PID Autotuner/3
  Closed-Loop PID Autotuner/3 -> Update PID Gains Z/1(PID Gains Z), Display/1
  Step1/1 -> Sum/2
  Step/1 -> Sum/1
  Sum/1 -> Gain1/1

== system MultirotorModel_Debugging/Inner Loop and Plant Model/High-FidelityModel/Plant Model/AC model/Drag Calculation/Drag Calc ==
  Density : Inport  Unit=kg/m^3
  vel : Inport  Port=2  Unit=m/s
  Dynamic Pressure : aerolibasang/Dynamic Pressure
  Gain : Gain  Gain=[.25 .25]
  Mux1 : Mux  Inputs=2
  Product : Product  Inputs=3  RndMeth=Zero
  diameter : Constant  Value=Vehicle.Airframe.diameter  SampleTime=0
  dragCoeff : Constant  Value=Vehicle.Airframe.Cdx  SampleTime=0
  drag : Outport  Unit=N  VectorParamsAs1DForOutWhenUnconnected=off
  wires:
  Product/1 -> drag/1
  dragCoeff/1 -> Product/3  "Cd"
  Dynamic Pressure/1 -> Product/1  "q"
  diameter/1 -> Gain/1, Mux1/2
  Mux1/1 -> Product/2  "S"
  Gain/1 -> Mux1/1
  vel/1 -> Dynamic Pressure/1
  Density/1 -> Dynamic Pressure/2

== system MultirotorModel_Debugging/Inner Loop and Plant Model/High-FidelityModel/Plant Model/AC model/Motor Forces and Torques/For Each Subsystem ==
  Vb : Inport  PortDimensions=3
  rho : Inport  Port=2  PortDimensions=1
  Omega : Inport  Port=3
  w : Inport  Port=4  Partition=on  PartitionDimension=2  PartitionWidth=1  PartitionOffset=0
  D : Inport  Port=5  Partition=on  PartitionDimension=2  PartitionWidth=1  PartitionOffset=0
  For Each : ForEach  DisableCoverage=on
  RotorDynamics : Subsystem  TreatAsAtomicUnit=on
      mask init:
      | aeroicon('aeroblk');
      settings: RTWFcnNameOpts=Use subsystem name  RTWFileNameOpts=Use function name
  Forces : Outport  ConcatenationDimension=2  VectorParamsAs1DForOutWhenUnconnected=off
  Moments : Outport  Port=2  ConcatenationDimension=2  VectorParamsAs1DForOutWhenUnconnected=off
  wires:
  RotorDynamics/1(Fxyz) -> Forces/1
  RotorDynamics/2(Mxyz) -> Moments/1
  Vb/1 -> RotorDynamics/1(Vb)
  Omega/1 -> RotorDynamics/2(pqr)
  rho/1 -> RotorDynamics/3(rho)
  D/1 -> RotorDynamics/5(Arm)
  w/1 -> RotorDynamics/4(w)

== system MultirotorModel_Debugging/Inner Loop and Plant Model/High-FidelityModel/Plant Model/AC model/Motor Forces and Torques/MotorsToW ==
  motors_datin : Inport
  Motordirections : Gain  Gain=[1 -1 1 -1]  ParamDataTypeStr=single  OutDataTypeStr=Inherit: Inherit via back propagation  SaturateOnIntegerOverflow=on
  Motordirections1 : Gain  Gain=[1 -1 1 -1]  ParamDataTypeStr=single  OutDataTypeStr=Inherit: Inherit via back propagation  SaturateOnIntegerOverflow=on
  Saturation5 : Saturate  UpperLimit=Vehicle.Motor.maxLimit  LowerLimit=Vehicle.Motor.minLimit  OutDataTypeStr=Inherit: Inherit via back propagation
  Signed Sqrt : Sqrt  Operator=signedSqrt  OutDataTypeStr=Inherit: Inherit via back propagation
  motorsToW2_Gain : Gain  Gain=Vehicle.Motor.commandToW2Gain  ParamDataTypeStr=single  OutDataTypeStr=Inherit: Inherit via back propagation  SaturateOnIntegerOverflow=on
  omegas_datout : Outport  VectorParamsAs1DForOutWhenUnconnected=off
  wires:
  motorsToW2_Gain/1 -> Signed Sqrt/1
  Motordirections/1 -> Saturation5/1
  Saturation5/1 -> Motordirections1/1
  Motordirections1/1 -> motorsToW2_Gain/1
  Signed Sqrt/1 -> omegas_datout/1
  motors_datin/1 -> Motordirections/1

== system MultirotorModel_Debugging/Inner Loop and Plant Model/High-FidelityModel/Plant Model/Bus setup/Generate GPS Data/Scale and Assemble GPS Data  ==
  Xe : Inport
  Ve : Inport  Port=2
  Angle Conversion1 : aerolibconvert2/Angle Conversion  IU=rad  OU=deg
  Bus Creator1 : BusCreator  Inputs=9  OutDataTypeStr=Bus: gps_raw_int  NonVirtualBus=on
      settings: InheritFromInputs=off
  Clock : Clock
      settings: AttributesFormatString=Decimation: %<Decimation>
  Data Type Conversion : DataTypeConversion  OutDataTypeStr=uint32  SaturateOnIntegerOverflow=off  RndMeth=Floor
  Demux1 : Demux  Outputs=3
  Demux2 : Demux  Outputs=2
  Embedded MATLAB Function1 : MATLAB Function  TreatAsAtomicUnit=on
  Fcn : Fcn  Expr=sqrt(u(1)^2+u(2)^2+u(3)^2)
  Flat Earth to LLA : FlatEarth2LLA  R=6378137  LL0=uavIC_latLon
  Gain : Gain  Gain=1e7  OutDataTypeStr=int32
  Gain1 : Gain  Gain=1e7  OutDataTypeStr=int32
  Gain2 : Gain  Gain=-1e3  OutDataTypeStr=int32
  Gain3 : Gain  Gain=1e2  OutDataTypeStr=uint16
  Gain4 : Gain  Gain=1e2  OutDataTypeStr=uint16
  Rate Transition1 : RateTransition  Commented=through  OutPortSampleTime=0.005
  Terminator : Terminator
  Zero level trust : Constant  Value=0
      settings: AttributesFormatString=%<Value>
  Zero level trust5 : Constant  Value=3  OutDataTypeStr=uint8
      settings: AttributesFormatString=%<Value>
  Zero level trust6 : Constant  Value=80  OutDataTypeStr=uint16
      settings: AttributesFormatString=%<Value>
  Zero level trust7 : Constant  Value=80  OutDataTypeStr=uint16
      settings: AttributesFormatString=%<Value>
  Out1 : Outport
  wires:
  Demux2/1 -> Gain/1
  Gain/1 -> Bus Creator1/3
  Gain4/1 -> Bus Creator1/9
  Demux2/2 -> Gain1/1
  Embedded MATLAB Function1/1(cog) -> Angle Conversion1/1
  Rate Transition1/1 -> Bus Creator1/1
  Zero level trust6/1 -> Bus Creator1/6
  Gain3/1 -> Bus Creator1/8
  Clock/1 -> Data Type Conversion/1
  Ve/1 -> Demux1/1, Fcn/1
  Zero level trust7/1 -> Bus Creator1/7
  Data Type Conversion/1 -> Rate Transition1/1
  Demux1/2 -> Embedded MATLAB Function1/2(Ve)
  Zero level trust5/1 -> Bus Creator1/2
  Demux1/1 -> Embedded MATLAB Function1/1(Vn)
  Flat Earth to LLA/1 -> Demux2/1  "gps_latLon"
  Gain2/1 -> Bus Creator1/5
  Fcn/1 -> Gain3/1  "gps_sog"
  Gain1/1 -> Bus Creator1/4
  Flat Earth to LLA/2 -> Gain2/1  "gps_h"
  Zero level trust/1 -> Flat Earth to LLA/2
  Angle Conversion1/1 -> Gain4/1  "gps_cog"
  Demux1/3 -> Terminator/1
  Xe/1 -> Flat Earth to LLA/1
  Bus Creator1/1 -> Out1/1

== system MultirotorModel_Debugging/Inner Loop and Plant Model/High-FidelityModel with Autotuning/Control System/Controller/Attitude Controller/Angle Loop Autotuning ==
  AngCtrl_out : Inport
  pitchroll_fdbk : Inport  Port=2
  Closed-Loop PID Autotuner : slctrl_autotuning/Closed-Loop PID Autotuner  PIDType=P  PIDForm=Parallel  TimeDomain=discrete-time  DiscreteTs=UAVSampleTime  TuningTs=0.2  UseTuningTs=off  IntegratorFormula=Forward Euler  FilterFormula=Forward Euler  ContinuousTs=0.02  Bandwidth=angControlTuning.wc  UseExternalWC=off  TargetPM=angControlTuning.pm  UseExternalPM=off  UseExternalAchievedPM=off  ExperimentMode=Superposition  PlantType=Stable  PlantSign=Positive  AmpSine=angControlTuning.sineAmp  UseExternalAmpSine=off  UseExternalFRD=off  UseExternalU0=off  UseCompanion=off  NotDeployTuningModule=off  UsePLCCoder=off  OutputMode=perturbation only  BlockDataType=single  UseExperimentGoodPort=off  UseConnectedPID=on  blockpath=[]  tunedP=0  tunedI=0  tunedD=0  tunedN=100  tunedPM=0  EstimationWindowSize=3  UseExternalTuningParams=off  SingleMultiRateVariant=SingleSamplingRate  NumEstimationPeriods=4  NumSettlingPeriods=2  NumOfPRBSPeriod=1  PRBSSignalOrder=12  ExperimentModeVariant=VariantSuperimposed  OutputChoice=VariantDonly  ConvergenceCalcVariant=ConvSuperpositionPRBSVariant
  Closed-Loop PID Autotuner1 : slctrl_autotuning/Closed-Loop PID Autotuner  PIDType=P  PIDForm=Parallel  TimeDomain=discrete-time  DiscreteTs=UAVSampleTime  TuningTs=0.2  UseTuningTs=off  IntegratorFormula=Forward Euler  FilterFormula=Forward Euler  ContinuousTs=0.02  Bandwidth=angControlTuning.wc  UseExternalWC=off  TargetPM=angControlTuning.pm  UseExternalPM=off  UseExternalAchievedPM=off  ExperimentMode=Superposition  PlantType=Stable  PlantSign=Positive  AmpSine=angControlTuning.sineAmp  UseExternalAmpSine=off  UseExternalFRD=off  UseExternalU0=off  UseCompanion=off  NotDeployTuningModule=off  UsePLCCoder=off  OutputMode=perturbation only  BlockDataType=single  UseExperimentGoodPort=off  UseConnectedPID=on  blockpath=[]  tunedP=0  tunedI=0  tunedD=0  tunedN=100  tunedPM=0  EstimationWindowSize=3  UseExternalTuningParams=off  SingleMultiRateVariant=SingleSamplingRate  NumEstimationPeriods=4  NumSettlingPeriods=2  NumOfPRBSPeriod=1  PRBSSignalOrder=12  ExperimentModeVariant=VariantSuperimposed  OutputChoice=VariantDonly  ConvergenceCalcVariant=ConvSuperpositionPRBSVariant
  Display : Display
  Display1 : Display
  Mux : Mux  Inputs=2
  Scope : Scope
      settings: ActiveDisplayYMinimum=99.18257  ActiveDisplayYMaximum=100.62707  DataLoggingVariableName=ScopeData9
  Scope1 : Scope
      settings: DataLoggingVariableName=ScopeData10
  Selector : Selector  InputPortWidth=2  IndexOptions=Index vector (dialog)  Indices=1  OutputSizes=1
  Selector1 : Selector  InputPortWidth=2  IndexOptions=Index vector (dialog)  Indices=1  OutputSizes=1
  Selector2 : Selector  InputPortWidth=2  IndexOptions=Index vector (dialog)  Indices=2  OutputSizes=1
  Selector3 : Selector  InputPortWidth=2  IndexOptions=Index vector (dialog)  Indices=2  OutputSizes=1
  Step : Step  Time=angControlTuning.startExpRoll  SampleTime=UAVSampleTime
  Step1 : Step  Time=angControlTuning.stopExpRoll  After=-1  SampleTime=UAVSampleTime
  Step2 : Step  Time=angControlTuning.startExpPitch  SampleTime=UAVSampleTime
  Step3 : Step  Time=angControlTuning.stopExpPitch  After=-1  SampleTime=UAVSampleTime
  Sum : Sum  Inputs=|++
  Sum1 : Sum  Inputs=|++
  Update PID Gains : Subsystem
  pitchroll_perturb : Outport
  wires:
  Closed-Loop PID Autotuner1/3 -> Update PID Gains/4(PID Gains roll), Display1/1
  Closed-Loop PID Autotuner/3 -> Update PID Gains/1(PID Gains pitch), Display/1
  AngCtrl_out/1 -> Selector2/1, Selector/1
  pitchroll_fdbk/1 -> Selector3/1, Selector1/1
  Selector/1 -> Closed-Loop PID Autotuner/1
  Selector1/1 -> Closed-Loop PID Autotuner/2
  Sum/1 -> Update PID Gains/2(start/stop pitch), Closed-Loop PID Autotuner/3
  Step2/1 -> Sum/1
  Step3/1 -> Sum/2
  Closed-Loop PID Autotuner/2 -> Scope/1
  Mux/1 -> pitchroll_perturb/1
  Closed-Loop PID Autotuner/1 -> Mux/1
  Selector2/1 -> Closed-Loop PID Autotuner1/1
  Selector3/1 -> Closed-Loop PID Autotuner1/2
  Step1/1 -> Sum1/2
  Step/1 -> Sum1/1
  Sum1/1 -> Update PID Gains/3(start/stop roll), Closed-Loop PID Autotuner1/3
  Closed-Loop PID Autotuner1/2 -> Scope1/1
  Closed-Loop PID Autotuner1/1 -> Mux/2

== system MultirotorModel_Debugging/Inner Loop and Plant Model/High-FidelityModel with Autotuning/Control System/Controller/Attitude Controller/Angular Velocity Loop Autotuning ==
  AngVelCtrl_out : Inport
  pitchrollrate_fdbk : Inport  Port=2
  Closed-Loop PID Autotuner : slctrl_autotuning/Closed-Loop PID Autotuner  PIDType=PIDF  PIDForm=Parallel  TimeDomain=discrete-time  DiscreteTs=UAVSampleTime  TuningTs=0.2  UseTuningTs=off  IntegratorFormula=Forward Euler  FilterFormula=Forward Euler  ContinuousTs=0.02  Bandwidth=angRateControlTuning.wc  UseExternalWC=off  TargetPM=angRateControlTuning.pm  UseExternalPM=off  UseExternalAchievedPM=off  ExperimentMode=Superposition  PlantType=Stable  PlantSign=Positive  AmpSine=angRateControlTuning.sineAmp  UseExternalAmpSine=off  UseExternalFRD=off  UseExternalU0=off  UseCompanion=off  NotDeployTuningModule=off  UsePLCCoder=off  OutputMode=perturbation only  BlockDataType=single  UseExperimentGoodPort=off  UseConnectedPID=on  blockpath=[]  tunedP=0  tunedI=0  tunedD=0  tunedN=100  tunedPM=0  EstimationWindowSize=3  UseExternalTuningParams=off  SingleMultiRateVariant=SingleSamplingRate  NumEstimationPeriods=4  NumSettlingPeriods=2  NumOfPRBSPeriod=1  PRBSSignalOrder=12  ExperimentModeVariant=VariantSuperimposed  OutputChoice=VariantDonly  ConvergenceCalcVariant=ConvSuperpositionPRBSVariant
  Closed-Loop PID Autotuner1 : slctrl_autotuning/Closed-Loop PID Autotuner  PIDType=PIDF  PIDForm=Parallel  TimeDomain=discrete-time  DiscreteTs=UAVSampleTime  TuningTs=0.2  UseTuningTs=off  IntegratorFormula=Forward Euler  FilterFormula=Forward Euler  ContinuousTs=0.02  Bandwidth=angRateControlTuning.wc  UseExternalWC=off  TargetPM=angRateControlTuning.pm  UseExternalPM=off  UseExternalAchievedPM=off  ExperimentMode=Superposition  PlantType=Stable  PlantSign=Positive  AmpSine=angRateControlTuning.sineAmp  UseExternalAmpSine=off  UseExternalFRD=off  UseExternalU0=off  UseCompanion=off  NotDeployTuningModule=off  UsePLCCoder=off  OutputMode=perturbation only  BlockDataType=single  UseExperimentGoodPort=off  UseConnectedPID=on  blockpath=[]  tunedP=0  tunedI=0  tunedD=0  tunedN=100  tunedPM=0  EstimationWindowSize=3  UseExternalTuningParams=off  SingleMultiRateVariant=SingleSamplingRate  NumEstimationPeriods=4  NumSettlingPeriods=2  NumOfPRBSPeriod=1  PRBSSignalOrder=12  ExperimentModeVariant=VariantSuperimposed  OutputChoice=VariantDonly  ConvergenceCalcVariant=ConvSuperpositionPRBSVariant
  Display : Display
  Display1 : Display
  Mux : Mux  Inputs=2
  Scope : Scope
      settings: ActiveDisplayYMinimum=99.18257  ActiveDisplayYMaximum=100.62707  DataLoggingVariableName=ScopeData9
  Scope1 : Scope
      settings: DataLoggingVariableName=ScopeData10
  Selector : Selector  InputPortWidth=2  IndexOptions=Index vector (dialog)  Indices=1  OutputSizes=1
  Selector1 : Selector  InputPortWidth=2  IndexOptions=Index vector (dialog)  Indices=1  OutputSizes=1
  Selector2 : Selector  InputPortWidth=2  IndexOptions=Index vector (dialog)  Indices=2  OutputSizes=1
  Selector3 : Selector  InputPortWidth=2  IndexOptions=Index vector (dialog)  Indices=2  OutputSizes=1
  Step : Step  Time=angRateControlTuning.startExpRoll  SampleTime=UAVSampleTime
  Step1 : Step  Time=angRateControlTuning.stopExpRoll  After=-1  SampleTime=UAVSampleTime
  Step2 : Step  Time=angRateControlTuning.startExpPitch  SampleTime=UAVSampleTime
  Step3 : Step  Time=angRateControlTuning.stopExpPitch  After=-1  SampleTime=UAVSampleTime
  Sum : Sum  Inputs=|++
  Sum1 : Sum  Inputs=|++
  Update PID Gains : Subsystem
  pitchrollrate_perturb : Outport
  wires:
  Closed-Loop PID Autotuner1/1 -> Mux/2
  Closed-Loop PID Autotuner1/2 -> Scope1/1
  Sum1/1 -> Update PID Gains/3(start/stop rollrate), Closed-Loop PID Autotuner1/3
  Step/1 -> Sum1/1
  Step1/1 -> Sum1/2
  Selector3/1 -> Closed-Loop PID Autotuner1/2
  Selector2/1 -> Closed-Loop PID Autotuner1/1
  Closed-Loop PID Autotuner/1 -> Mux/1
  Mux/1 -> pitchrollrate_perturb/1
  Closed-Loop PID Autotuner/2 -> Scope/1
  Step3/1 -> Sum/2
  Step2/1 -> Sum/1
  Sum/1 -> Update PID Gains/2(start/stop pitchrate), Closed-Loop PID Autotuner/3
  Selector1/1 -> Closed-Loop PID Autotuner/2
  Selector/1 -> Closed-Loop PID Autotuner/1
  pitchrollrate_fdbk/1 -> Selector1/1, Selector3/1
  AngVelCtrl_out/1 -> Selector/1, Selector2/1
  Closed-Loop PID Autotuner/3 -> Update PID Gains/1(PID Gains pitchrate), Display/1
  Closed-Loop PID Autotuner1/3 -> Update PID Gains/4(PID Gains rollrate), Display1/1
